simulink model "without-attack"  (R2018b)
settings: Solver=VariableStepAuto  StartTime=0.0  StopTime=10  RelTol=1e-3
settings Model: Creator=lenovo  LastModifiedBy=lenovo

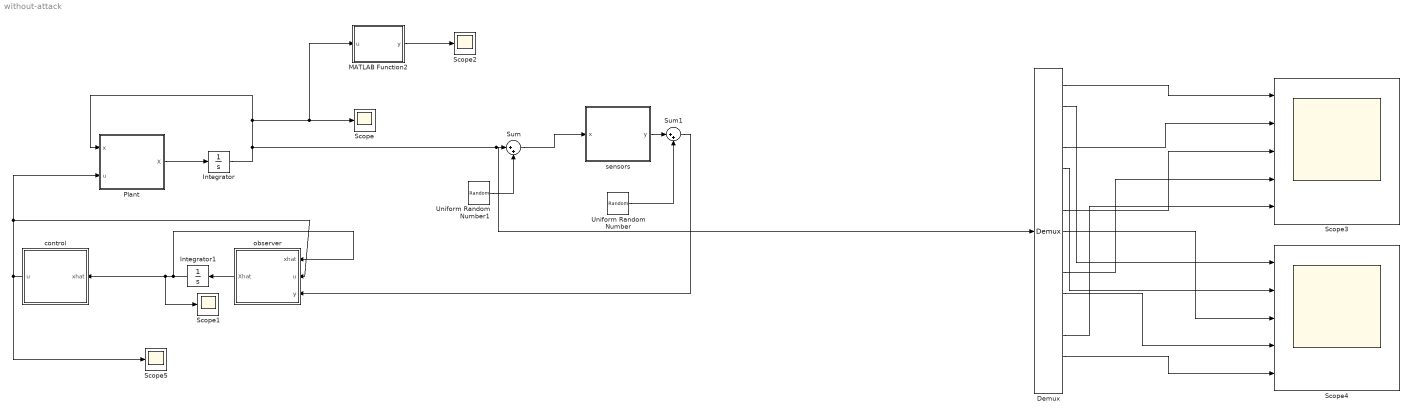
== system without-attack ==
  Demux : Demux  Outputs=15
  Integrator : Integrator  InitialCondition=10*[-7;-6;-5;-4;-3;-2;-1;0;1;2;3;4;5;6;7]
  Integrator1 : Integrator  InitialCondition=-10*[-7;-6;-5;-4;-3;-2;-1;0;1;2;3;4;5;6;7]
  MATLAB Function2 : MATLAB Function  TreatAsAtomicUnit=on
  Plant : MATLAB Function  TreatAsAtomicUnit=on
  Scope{,1..2,5} (4 alike) : Scope
  Scope3 : Scope  NumInputPorts=5
  Scope4 : Scope  NumInputPorts=5
  Sum : Sum  Inputs=|++
  Sum1 : Sum  Inputs=|++
  Uniform Random Number : UniformRandomNumber  Minimum=-0.01  Maximum=0.01  SampleTime=0.1
  Uniform Random Number1 : UniformRandomNumber  Minimum=-0.01  Maximum=0.01  SampleTime=0.1
  control : MATLAB Function  TreatAsAtomicUnit=on
  observer : MATLAB Function  TreatAsAtomicUnit=on
  sensors : MATLAB Function  TreatAsAtomicUnit=on
  wires:
  control/1(u) -> Plant/2(u), observer/2(u), Scope5/1
  observer/1(Xhat) -> Integrator1/1
  Integrator1/1 -> Scope1/1, control/1(xhat), observer/1(xhat)
  Plant/1(X) -> Integrator/1
  MATLAB Function2/1(y) -> Scope2/1
  sensors/1(y) -> Sum1/1
  Uniform Random Number1/1 -> Sum/2
  Sum/1 -> sensors/1(x)
  Sum1/1 -> observer/3(y)
  Uniform Random Number/1 -> Sum1/2
  Demux/10 -> Scope3/4
  Integrator/1 -> Demux/1, Sum/1, Plant/1(x), MATLAB Function2/1(u), Scope/1
  Demux/1 -> Scope3/1
  Demux/2 -> Scope4/1
  Demux/13 -> Scope3/5
  Demux/7 -> Scope3/3
  Demux/8 -> Scope4/3
  Demux/5 -> Scope4/2
  Demux/4 -> Scope3/2
  Demux/11 -> Scope4/4
  Demux/14 -> Scope4/5

== matlab function without-attack/control ==
  data: xhat input; u output
function u = fcn(xhat)
A=[ 1.049     0.03183    -0.02926
     0.01347       1.023  -0.0001932
  -0.0007729     -0.1155      0.9048];
B=[0.2026  6.946e-05
   -0.1504     0.1012
  0.008724    0.08931 ];
L=[ 1 0 0 0 -1; -1 1 0 0 0; -1 0 1 0 0; 0 -1 0 1 0; 0 -1 -1 -1 3];
A0=kron(eye(5),A);
B0=kron(eye(5),B);
z=kron(L,eye(3));
Q=z'*eye(15)*z;

q1=[1.9115   -1.1429    0.4148    0.0000    0.0000   -0.0000    0.0000    0.0000   -0.0000
    3.0186    4.4625   -0.5557   -0.0000   -0.0000    0.0000   -0.0000   -0.0000    0.0000
    0.0000    0.0000   -0.0000    1.9115   -1.1429    0.4148    0.0000    0.0000   -0.0000
   -0.0000   -0.0000    0.0000    3.0186    4.4625   -0.5557   -0.0000   -0.0000    0.0000
    0.0000    0.0000   -0.0000    0.0000    0.0000   -0.0000    1.9115   -1.1429    0.4148
   -0.0000   -0.0000    0.0000   -0.0000   -0.0000    0.0000    3.0186    4.4625   -0.5557
    0.0000    0.0000   -0.0000    0.0000    0.0000    0.0000    0.0000    0.0000   -0.0000
    0.0000    0.0000   -0.0000    0.0000    0.0000   -0.0000   -0.0000   -0.0000    0.0000
    0.0000    0.0000   -0.0000   -0.0000   -0.0000    0.0000   -0.0000   -0.0000    0.0000
    0.0000    0.0000   -0.0000    0.0000    0.0000   -0.0000    0.0000    0.0000   -0.0000
];
q2=[-0.0000   -0.0000    0.0000   -0.0000   -0.0000    0.0000
    0.0000    0.0000   -0.0000    0.0000    0.0000    0.0000
    0.0000    0.0000   -0.0000   -0.0000   -0.0000    0.0000
   -0.0000   -0.0000    0.0000    0.0000    0.0000   -0.0000
    0.0000    0.0000   -0.0000    0.0000    0.0000   -0.0000
   -0.0000   -0.0000    0.0000    0.0000    0.0000   -0.0000
    1.9115   -1.1429    0.4148   -0.0000   -0.0000    0.0000
    3.0186    4.4625   -0.5557   -0.0000   -0.0000    0.0000
    0.0000    0.0000   -0.0000    1.9115   -1.1429    0.4148
   -0.0000   -0.0000    0.0000    3.0186    4.4625   -0.5557
];
% K=[    1.9115   -1.1429    0.4148
%     3.0186    4.4625   -0.5557];
K=[q1 q2];
u=-K*xhat;

== matlab function without-attack/Plant ==
  data: x input; X output; u input
function X = fcn(x,u)
A=[.48 .29 -.3;.13 .23 0;0 -1.2 -1];
B=[2 0;-1.5 1; 0 1];
A0=kron(eye(5),A);
B0=kron(eye(5),B);
X =A0*x+B0*u;

== matlab function without-attack/sensors ==
  data: x input; y output
function y = fcn(x)
C=eye(3);
C0=kron(eye(5),C);
y=C0*x;

== matlab function without-attack/observer ==
  data: xhat input; u input; Xhat output; y input
function Xhat = fcn(xhat,u,y)
A=[.48 .29 -.3;.13 .23 0;0 -1.2 -1];
B=[2 0;-1.5 1; 0 1];
C=eye(3);
G=[ 5.0468    1.5160   -0.5215
    1.5160    1.8633   -0.6870
   -0.5215   -0.6870    1.1919];
C0=kron(eye(5),C);
A0=kron(eye(5),A);
B0=kron(eye(5),B);
G0=kron(eye(5),G);
yhat=C0*xhat;
Xhat=A0*xhat+B0*u+G0*(y-yhat);

== matlab function without-attack/MATLAB Function2 ==
  data: u input; y output
function y = fcn(u)
y=norm(u);
